simulink model "sampleModel280"  (R2021b)
settings: Solver=VariableStepAuto  StartTime=0.0  StopTime=10.0  RelTol=1e-3
undefined symbols (not defined in the file or in its folder): DiscIntNeverNeededParam, Newton, Raphson
libraries: simulink x14, slpidlib x1
settings Model: Creator=user  LastModifiedBy=user

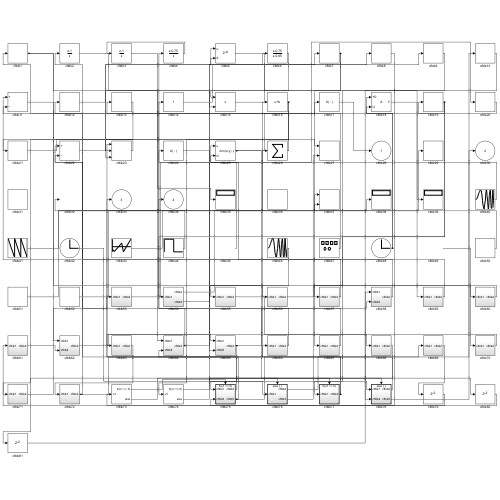
[thumbnail: Simulink's stored preview of the top-level diagram]
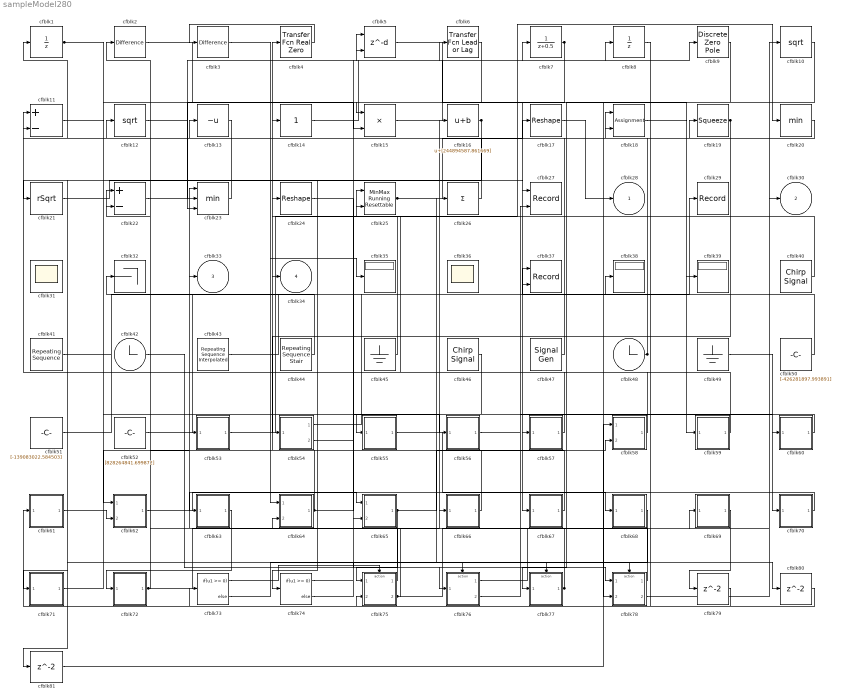
== system sampleModel280 ==
  cfblk1 : UnitDelay  HasFrameUpgradeWarning=on
  cfblk10 : Sqrt  SaturateOnIntegerOverflow=on
  cfblk11 : Sum  Inputs=+-
  cfblk12 : Sqrt  SaturateOnIntegerOverflow=on
  cfblk13 : UnaryMinus
  cfblk14 : simulink/Math Operations/Slider Gain  gain=1  low=0  high=2
  cfblk15 : Product
  cfblk16 : Bias  Bias=[244894587.861669]
  cfblk17 : Reshape
  cfblk18 : Assignment  DiagnosticForDimensions=Warning  IndexOptions=Index vector (dialog)  Indices=1  OutputSizes=1
  cfblk19 : Squeeze
  cfblk2 : simulink/Discrete/Difference  ICPrevInput=0.0  OutMin=[]  OutMax=[]  OutDataTypeStr=Inherit: Inherit via back propagation  OutDataType=fixdt(1, 16)  OutScaling=2^-10  DoSatur=off
  cfblk20 : MinMax
  cfblk21 : Sqrt  Operator=rSqrt  AlgorithmType=Newton-Raphson  SaturateOnIntegerOverflow=on
  cfblk22 : Sum  Inputs=+-
  cfblk23 : MinMax  Inputs=3
  cfblk24 : Reshape
  cfblk25 : simulink/Math Operations/MinMax Running Resettable  Function=min  vinit=0.0
  cfblk26 : Sum  Inputs=+
  cfblk27 : Record  FileSettingsInternal="{\"entries\":[{\"content\":{\"excelSettings\":{\"content\":{},\"type\":\"Streamout.ExcelSettings\"}},\"type\":\"Streamout.FileSettingStorage\",\"uuid\":\"01a86b24-10fd-47b5-8f86-b590ee2283c4\"}],\"packageUris\":[\"http://schema.mathworks.com/mf0/streamout_blocks/R2020a\"],\"version\":\"1.0\"}"  Layout=[1 1]  SignalsInternal="{\"entries\":[{\"content\":{\"signals\":[{\"content\":{\"blockPath\":[\"sampleModel280/cfblk27\"],\"channel\":[],\"dimensions\":[1],\"domain\":\"sampleModel280/cfblk27\",\"lineColor\":\"#a2142f\",\"plots\":[1],\"port\":1,\"sid\":[\"\"],\"signalID\":11869,\"signalName\":\"cfblk21\"},\"type\":\"RecordBlkView.Signal\",\"uuid\":\"a0fc44e3-e2e4-42ff-bb3b-f537f22ba603\"},{\"content\":{\"blockPath\":[\"sampleModel280/cfblk27\"],\"channel\":[],\"dimensions\":[1],\"domain\":\"sampleModel280/cfblk27\",\"lineColor\":\"#139fff\",\"plots\":[1],\"port\":2,\"sid\":[\"\"],\"signalID\":11873,\"signalName\":\"cfblk76:2\"},\"type\":\"RecordBlkView.Signal\",\"uuid\":\"77bcc749-ff83-4f0f-aafb-09d3bf5905dd\"}]},\"type\":\"RecordBlkView.InputSignals\",\"uuid\":\"96dfc8e1-6c66-4ba5-9853-10110527c52c\"}],\"packageUris\":[\"http://schema.mathworks.com/mf0/streamout_blocks/R2020a\"],\"version\":\"1.0\"}"  VisualizationBindings="{\"xyplotplugin\":{\"info\":[{\"series\":[{\"bindingParametersList\":[{\"parameter\":\"X-Axis\",\"signalID\":11869,\"signalName\":\"cfblk21\"},{\"parameter\":\"Y-Axis\",\"signalID\":11873,\"signalName\":\"cfblk76:2\"}],\"seriesID\":38376}],\"subplotID\":1}]}}"  CompatibilityTag=XY
  cfblk29 : Record  FileSettingsInternal="{\"entries\":[{\"content\":{\"excelSettings\":{\"content\":{},\"type\":\"Streamout.ExcelSettings\"}},\"type\":\"Streamout.FileSettingStorage\",\"uuid\":\"e8b19c5e-8c0f-47fc-b4c9-298200dd95d7\"}],\"packageUris\":[\"http://schema.mathworks.com/mf0/streamout_blocks/R2020a\"],\"version\":\"1.0\"}"  SignalsInternal="{\"entries\":[{\"content\":{\"signals\":[{\"content\":{\"blockPath\":[\"sampleModel280/cfblk29\"],\"channel\":[],\"dimensions\":[1],\"domain\":\"sampleModel280/cfblk29\",\"lineColor\":\"#edb120\",\"plots\":[1],\"port\":1,\"sid\":[\"\"],\"signalID\":11881,\"signalName\":\"cfblk51\"},\"type\":\"RecordBlkView.Signal\",\"uuid\":\"65e0956e-956d-4622-b740-1f07b225f85c\"}]},\"type\":\"RecordBlkView.InputSignals\",\"uuid\":\"866c25ee-dbf6-4b5f-85e6-0975c442b7af\"}],\"packageUris\":[\"http://schema.mathworks.com/mf0/streamout_blocks/R2020a\"],\"version\":\"1.0\"}"  VisualizationBindings="{\"sparklinesplugin\":{\"info\":[{\"bindingParametersList\":[],\"subplotID\":1}]}}"
  cfblk3 : simulink/Discrete/Difference  ICPrevInput=0.0  OutMin=[]  OutMax=[]  OutDataTypeStr=Inherit: Inherit via back propagation  OutDataType=fixdt(1, 16)  OutScaling=2^-10  DoSatur=off
  cfblk31 : Scope
      settings: Floating=on
  cfblk32 : Terminator
  cfblk35 : Display
  cfblk36 : Scope
      settings: Floating=on
  cfblk37 : Record  FileSettingsInternal="{\"entries\":[{\"content\":{\"excelSettings\":{\"content\":{},\"type\":\"Streamout.ExcelSettings\"}},\"type\":\"Streamout.FileSettingStorage\",\"uuid\":\"e62b4aea-36b7-4c87-85d7-a4ab9cb59138\"}],\"packageUris\":[\"http://schema.mathworks.com/mf0/streamout_blocks/R2020a\"],\"version\":\"1.0\"}"  Layout=[1 1]  SignalsInternal="{\"entries\":[{\"content\":{\"signals\":[{\"content\":{\"blockPath\":[\"sampleModel280/cfblk37\"],\"channel\":[],\"dimensions\":[1],\"domain\":\"sampleModel280/cfblk37\",\"lineColor\":\"#a2142f\",\"plots\":[1],\"port\":1,\"sid\":[\"\"],\"signalID\":11885,\"signalName\":\"cfblk43\"},\"type\":\"RecordBlkView.Signal\",\"uuid\":\"4226a702-03e0-4b16-abca-3234c63018e1\"},{\"content\":{\"blockPath\":[\"sampleModel280/cfblk37\"],\"channel\":[],\"dimensions\":[1],\"domain\":\"sampleModel280/cfblk37\",\"lineColor\":\"#139fff\",\"plots\":[1],\"port\":2,\"sid\":[\"\"],\"signalID\":11889,\"signalName\":\"cfblk50\"},\"type\":\"RecordBlkView.Signal\",\"uuid\":\"55b215cc-d555-4d8f-b13f-ef35d573dbbd\"}]},\"type\":\"RecordBlkView.InputSignals\",\"uuid\":\"d3c2a2c5-2de7-407e-9157-1018b6e42a97\"}],\"packageUris\":[\"http://schema.mathworks.com/mf0/streamout_blocks/R2020a\"],\"version\":\"1.0\"}"  VisualizationBindings="{\"xyplotplugin\":{\"info\":[{\"series\":[{\"bindingParametersList\":[{\"parameter\":\"X-Axis\",\"signalID\":11885,\"signalName\":\"cfblk43\"},{\"parameter\":\"Y-Axis\",\"signalID\":11889,\"signalName\":\"cfblk50\"}],\"seriesID\":28925}],\"subplotID\":1}]}}"  CompatibilityTag=XY
  cfblk38 : Display
  cfblk39 : Display
  cfblk4 : simulink/Discrete/Transfer Fcn Real Zero  ZeroZ=0.75  ICPrevInput=0.0  DoSatur=off
      settings: SourceProductBaseCode=SL
  cfblk40 : simulink/Sources/Chirp Signal  f1=[477583071.067130]  T=[170289565.158624]  f2=[-132189540.561952]
  cfblk41 : simulink/Sources/Repeating Sequence  rep_seq_t=[0 2]  rep_seq_y=[470306380.096808, -725988435.533882]
  cfblk42 : Clock
  cfblk43 : simulink/Sources/Repeating Sequence Interpolated  OutValues=[-280109527.984477, -640686721.339378, 480149620.737201, -658559004.004570, 983301595.274376]  TimeValues=[0 0.1 0.5 0.6 1].'  LookUpMeth=Interpolation-Use End Values  tsamp=0.01  OutMin=[]  OutMax=[]  OutDataTypeStr=double  OutputDataTypeScalingMode=double  OutDataType=fixdt(0,8)  OutScaling=2^-10
  cfblk44 : simulink/Sources/Repeating Sequence Stair  OutValues=[152099642.248450, 137848680.236196]  tsamp=-1  OutMin=[]  OutMax=[]  OutDataTypeStr=double  OutputDataTypeScalingMode=double  OutDataType=fixdt(0,8)  ConRadixGroup=Best Precision: Vector-wise  OutScaling=2^-12
  cfblk45 : Ground
  cfblk46 : simulink/Sources/Chirp Signal  f1=[-254697657.951645]  T=[-710962001.298007]  f2=[-290174974.004187]
  cfblk47 : SignalGenerator  WaveForm=square  Amplitude=[315229153.492773]  Units=rad/sec
  cfblk48 : Clock
  cfblk49 : Ground
  cfblk5 : Delay  DelayLengthSource=Input port  SampleTime=1
      settings: InputPortMap=u0,p1
  cfblk50 : Constant  Value=[-426281897.993891]  SampleTime=1
  cfblk51 : Constant  Value=[-139083022.584503]  SampleTime=1
  cfblk52 : Constant  Value=[828264841.699872]  SampleTime=1
  cfblk53 : Subsystem
  cfblk54 : Subsystem
  cfblk55 : Subsystem
  cfblk56 : Subsystem
  cfblk57 : Subsystem
  cfblk58 : Subsystem
  cfblk59 : Subsystem
  cfblk6 : simulink/Discrete/Transfer Fcn Lead or Lag  PoleZ=0.95  ZeroZ=0.75  ICPrevOutput=0.0  ICPrevInput=0.0  DoSatur=off
      settings: SourceProductBaseCode=SL
  cfblk60 : Subsystem
  cfblk61 : Subsystem
  cfblk62 : Subsystem
  cfblk63 : Subsystem
  cfblk64 : Subsystem
  cfblk65 : Subsystem
  cfblk66 : Subsystem
  cfblk67 : Subsystem
  cfblk68 : Subsystem
  cfblk69 : Subsystem
  cfblk7 : DiscreteTransferFcn  SampleTime=1
  cfblk70 : Subsystem
  cfblk71 : Subsystem
  cfblk72 : Subsystem
  cfblk73 : If  IfExpression=u1 >= 0  SampleTime=1
  cfblk74 : If  IfExpression=u1 >= 0  SampleTime=1
  cfblk75 : Subsystem  TreatAsAtomicUnit=on
  cfblk76 : Subsystem  TreatAsAtomicUnit=on
  cfblk77 : Subsystem  TreatAsAtomicUnit=on
  cfblk78 : Subsystem  TreatAsAtomicUnit=on
  cfblk79 : Delay  SampleTime=1
  cfblk8 : UnitDelay  HasFrameUpgradeWarning=on
  cfblk80 : Delay  SampleTime=1
  cfblk81 : Delay  SampleTime=1
  cfblk9 : DiscreteZeroPole  Poles=[0 0.5]  Gain=1
  cfblk28 : Outport
  cfblk30 : Outport  Port=2
  cfblk33 : Outport  Port=3
  cfblk34 : Outport  Port=4
  wires:
  cfblk26/1 -> cfblk13/1
  cfblk78/1(cfblk2) -> cfblk23/1
  cfblk17/1 -> cfblk28/1
  cfblk7/1 -> cfblk67/1(cfblk1), cfblk15/1
  cfblk53/1(cfblk2) -> cfblk20/1
  cfblk15/1 -> cfblk8/1
  cfblk64/1(cfblk2) -> cfblk4/1, cfblk9/1
  cfblk42/1 -> cfblk78/1(cfblk1)
  cfblk62/1(cfblk2) -> cfblk65/1(cfblk1)
  cfblk44/1 -> cfblk32/1
  cfblk75/1(cfblk2) -> cfblk33/1
  cfblk20/1 -> cfblk19/1
  cfblk52/1 -> cfblk14/1
  cfblk63/1(cfblk2) -> cfblk72/1(cfblk1)
  cfblk8/1 -> cfblk61/1(cfblk1)
  cfblk54/1(cfblk2) -> cfblk38/1
  cfblk65/1(cfblk2) -> cfblk75/1(cfblk1), cfblk58/2(cfblk5)
  cfblk58/1(cfblk2) -> cfblk12/1
  cfblk13/1 -> cfblk71/1(cfblk1)
  cfblk2/1 -> cfblk64/1(cfblk1)
  cfblk21/1 -> cfblk27/1
  cfblk67/1(cfblk2) -> cfblk34/1
  cfblk3/1 -> cfblk35/1
  cfblk57/1(cfblk2) -> cfblk25/1
  cfblk25/1 -> cfblk17/1, cfblk80/1
  cfblk19/1 -> cfblk54/1(cfblk1), cfblk18/2, cfblk77/1(cfblk1)
  cfblk70/1(cfblk2) -> cfblk63/1(cfblk1)
  cfblk72/1(cfblk2) -> cfblk16/1, cfblk22/2
  cfblk71/1(cfblk2) -> cfblk53/1(cfblk1)
  cfblk4/1 -> cfblk3/1
  cfblk59/1(cfblk2) -> cfblk11/1
  cfblk55/1(cfblk2) -> cfblk68/1(cfblk1)
  cfblk16/1 -> cfblk74/1, cfblk23/3
  cfblk10/1 -> cfblk78/2(cfblk4)
  cfblk40/1 -> cfblk25/2
  cfblk11/1 -> cfblk56/1(cfblk1)
  cfblk49/1 -> cfblk70/1(cfblk1)
  cfblk9/1 -> cfblk57/1(cfblk1)
  cfblk22/1 -> cfblk5/1
  cfblk45/1 -> cfblk24/1
  cfblk66/1(cfblk2) -> cfblk22/1
  cfblk75/2(cfblk5) -> cfblk69/1(cfblk1), cfblk64/2(cfblk4)
  cfblk5/1 -> cfblk59/1(cfblk1)
  cfblk23/1 -> cfblk21/1
  cfblk14/1 -> cfblk7/1
  cfblk51/1 -> cfblk29/1
  cfblk60/1(cfblk2) -> cfblk55/1(cfblk1)
  cfblk47/1 -> cfblk11/2
  cfblk56/1(cfblk2) -> cfblk60/1(cfblk1)
  cfblk24/1 -> cfblk76/1(cfblk1)
  cfblk46/1 -> cfblk65/2(cfblk5)
  cfblk54/2(cfblk5) -> cfblk6/1
  cfblk41/1 -> cfblk26/1
  cfblk43/1 -> cfblk37/1
  cfblk18/1 -> cfblk39/1
  cfblk1/1 -> cfblk62/1(cfblk1), cfblk15/2
  cfblk61/1(cfblk2) -> cfblk62/2(cfblk4)
  cfblk78/2(cfblk5) -> cfblk30/1
  cfblk50/1 -> cfblk37/2
  cfblk48/1 -> cfblk1/1, cfblk18/1
  cfblk6/1 -> cfblk23/2
  cfblk77/1(cfblk2) -> cfblk2/1, cfblk66/1(cfblk1)
  cfblk12/1 -> cfblk5/2
  cfblk76/1(cfblk2) -> cfblk10/1
  cfblk76/2(cfblk3) -> cfblk27/2
  cfblk73/1 -> cfblk75/Action
  cfblk73/2 -> cfblk76/Action
  cfblk74/1 -> cfblk77/Action
  cfblk74/2 -> cfblk78/Action
  cfblk69/1(cfblk2) -> cfblk79/1
  cfblk79/1 -> cfblk75/2(cfblk4)
  cfblk80/1 -> cfblk73/1
  cfblk68/1(cfblk2) -> cfblk81/1
  cfblk81/1 -> cfblk58/1(cfblk1)

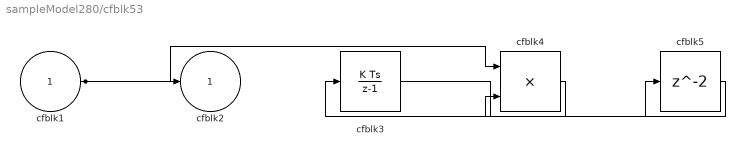
== system sampleModel280/cfblk53 ==
  cfblk1 : Inport
  cfblk3 : DiscreteIntegrator  ICPrevOutput=DiscIntNeverNeededParam  ICPrevScaledInput=DiscIntNeverNeededParam
  cfblk4 : Product  Inputs=**
  cfblk5 : Delay  SampleTime=1
  cfblk2 : Outport
  wires:
  cfblk1/1 -> cfblk4/1, cfblk2/1
  cfblk4/1 -> cfblk3/1
  cfblk3/1 -> cfblk5/1
  cfblk5/1 -> cfblk4/2

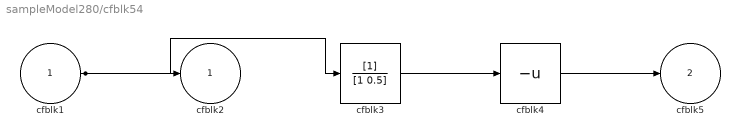
== system sampleModel280/cfblk54 ==
  cfblk1 : Inport
  cfblk3 : DiscreteFilter  SampleTime=1
  cfblk4 : UnaryMinus
  cfblk2 : Outport
  cfblk5 : Outport  Port=2
  wires:
  cfblk1/1 -> cfblk3/1, cfblk2/1
  cfblk3/1 -> cfblk4/1
  cfblk4/1 -> cfblk5/1

== system sampleModel280/cfblk55 ==
  cfblk1 : Inport
  cfblk3 : Assignment  DiagnosticForDimensions=Warning  IndexOptions=Index vector (dialog)  Indices=1  OutputSizes=1
  cfblk2 : Outport
  wires:
  cfblk1/1 -> cfblk3/1, cfblk3/2
  cfblk3/1 -> cfblk2/1

== system sampleModel280/cfblk56 ==
  cfblk1 : Inport
  cfblk3 : slpidlib/PID Controller  Controller=PID  Form=Parallel  TimeDomain=Discrete-time  UseExternalTs=off  SampleTime=1  IntegratorMethod=Forward Euler  FilterMethod=Forward Euler  ControllerParametersSource=internal  P=1  I=1  D=0  UseFilter=on  N=100  TunerSelectOption=Transfer Function Based (PID Tuner App)  InitialConditionSource=internal  InitialConditionForIntegrator=0  InitialConditionForFilter=0  DifferentiatorICPrevScaledInput=0  ExternalReset=none  TrackingMode=off  Kt=1  LimitOutput=off  SatLimitsSource=internal  UpperSaturationLimit=inf  LowerSaturationLimit=-inf  LinearizeAsGain=off  AntiWindupMode=none  Kb=1  POutMin=[]  POutMax=[]  IOutMin=[]  IOutMax=[]  DOutMin=[]  DOutMax=[]  NOutMin=[]  NOutMax=[]  SumOutMin=[]  SumOutMax=[]  SaturationOutMin=[]  SaturationOutMax=[]  PParamMin=[]  PParamMax=[]  IParamMin=[]  IParamMax=[]  DParamMin=[]  DParamMax=[]  NParamMin=[]  NParamMax=[]  KbParamMin=[]  KbParamMax=[]  KtParamMin=[]  KtParamMax=[]  KbOutMin=[]  KbOutMax=[]  KtOutMin=[]  KtOutMax=[]  IntegratorOutMin=[]  IntegratorOutMax=[]  FilterOutMin=[]  FilterOutMax=[]  SumI1OutMin=[]  SumI1OutMax=[]  SumI2OutMin=[]  SumI2OutMax=[]  SumI3OutMin=[]  SumI3OutMax=[]  SumI4OutMin=[]  SumI4OutMax=[]  SumDOutMin=[]  SumDOutMax=[]  DifferentiatorOutMin=[]  DifferentiatorOutMax=[]  FilterDiffOutCoefMin=[]  FilterDiffOutCoefMax=[]  ReciprocalOutMin=[]  ReciprocalOutMax=[]  SumDenOutMin=[]  SumDenOutMax=[]  SumNumOutMin=[]  SumNumOutMax=[]  DivideOutMin=[]  DivideOutMax=[]  UdiffTsProdOutMin=[]  UdiffTsProdOutMax=[]  NTsProdOutMin=[]  NTsProdOutMax=[]  UintegralTsProdOutMin=[]  UintegralTsProdOutMax=[]  UngainTsProdOutMin=[]  UngainTsProdOutMax=[]  IntegratorContinuousStateAttributes=''  IntegratorStateMustResolveToSignalObject=off  IntegratorRTWStateStorageClass=Auto  FilterContinuousStateAttributes=''  FilterStateMustResolveToSignalObject=off  FilterRTWStateStorageClass=Auto  ParallelPVariant=InternalParameters  IdealPVariant=Disabled  IVariant=InternalParameters  DVariant=InternalParameters  IntegratorVariant=Discrete  SatVariant=Disabled  AWVariant=Passthrough  PCopyVariant=Disabled  TRVariant=Disabled  FdbkBlocksVariant=Forward  IdealPFdbkVariant=Disabled  SatFdbkVariant=Disabled  DerivativeFilterVariant=ForwardEulerFilter  NVariant=InternalParameters  NCopyVariant=Disabled  FilterICVariant=InternalICsFilter  IntegratorICVariant=InternalICs  ExternalResetVariant=Disabled  TRSumVariant=Passthrough  SumFdbkVariant=Disabled  SumVariant=Sum_PID  TsampFilterVariant=InternalTs  TsampNgainVariant=Passthrough  TsampIntegralVariant=Passthrough  ExternalSaturationOutDataTypeStr=Inherit: Same as second input
  cfblk4 : Product  Inputs=*
  cfblk2 : Outport
  wires:
  cfblk4/1 -> cfblk2/1
  cfblk3/1 -> cfblk4/1
  cfblk1/1 -> cfblk3/1

== system sampleModel280/cfblk57 ==
  cfblk1 : Inport
  cfblk3 : DotProduct  InputSameDT=on  OutDataTypeStr=Inherit: Inherit via internal rule
  cfblk2 : Outport
  wires:
  cfblk1/1 -> cfblk3/1, cfblk3/2
  cfblk3/1 -> cfblk2/1

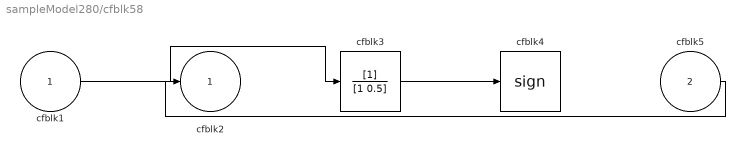
== system sampleModel280/cfblk58 ==
  cfblk1 : Inport
  cfblk5 : Inport  Port=2
  cfblk3 : DiscreteFilter  SampleTime=1
  cfblk4 : Signum
  cfblk2 : Outport
  wires:
  cfblk3/1 -> cfblk4/1
  cfblk1/1 -> cfblk3/1
  cfblk5/1 -> cfblk2/1

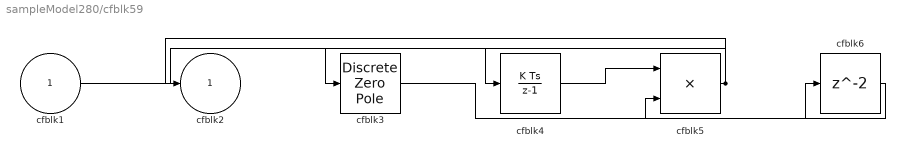
== system sampleModel280/cfblk59 ==
  cfblk1 : Inport
  cfblk3 : DiscreteZeroPole  Poles=[0 0.5]  Gain=1
  cfblk4 : DiscreteIntegrator  ICPrevOutput=DiscIntNeverNeededParam  ICPrevScaledInput=DiscIntNeverNeededParam
  cfblk5 : Product  Inputs=**
  cfblk6 : Delay  SampleTime=1
  cfblk2 : Outport
  wires:
  cfblk1/1 -> cfblk4/1
  cfblk4/1 -> cfblk5/1
  cfblk5/1 -> cfblk2/1, cfblk3/1
  cfblk3/1 -> cfblk6/1
  cfblk6/1 -> cfblk5/2

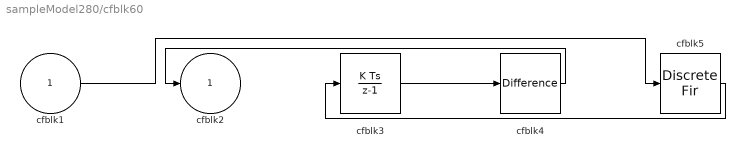
== system sampleModel280/cfblk60 ==
  cfblk1 : Inport
  cfblk3 : DiscreteIntegrator  ICPrevOutput=DiscIntNeverNeededParam  ICPrevScaledInput=DiscIntNeverNeededParam
  cfblk4 : simulink/Discrete/Difference  ICPrevInput=0.0  OutMin=[]  OutMax=[]  OutDataTypeStr=Inherit: Inherit via back propagation  OutDataType=fixdt(1, 16)  OutScaling=2^-10  DoSatur=off
  cfblk5 : DiscreteFir  SampleTime=1
  cfblk2 : Outport
  wires:
  cfblk3/1 -> cfblk4/1
  cfblk4/1 -> cfblk2/1
  cfblk5/1 -> cfblk3/1
  cfblk1/1 -> cfblk5/1

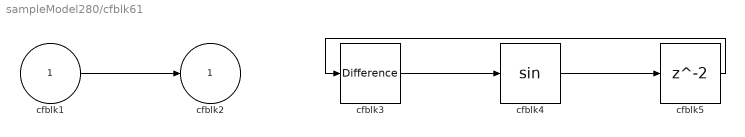
== system sampleModel280/cfblk61 ==
  cfblk1 : Inport
  cfblk3 : simulink/Discrete/Difference  ICPrevInput=0.0  OutMin=[]  OutMax=[]  OutDataTypeStr=Inherit: Inherit via back propagation  OutDataType=fixdt(1, 16)  OutScaling=2^-10  DoSatur=off
  cfblk4 : Trigonometry
  cfblk5 : Delay  SampleTime=1
  cfblk2 : Outport
  wires:
  cfblk3/1 -> cfblk4/1
  cfblk1/1 -> cfblk2/1
  cfblk4/1 -> cfblk5/1
  cfblk5/1 -> cfblk3/1

== system sampleModel280/cfblk62 ==
  cfblk1 : Inport
  cfblk4 : Inport  Port=2
  cfblk3 : Constant  Value=[452989492.075059]  SampleTime=1
  cfblk2 : Outport
  wires:
  cfblk4/1 -> cfblk2/1

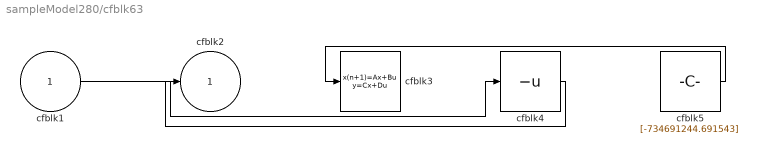
== system sampleModel280/cfblk63 ==
  cfblk1 : Inport
  cfblk3 : DiscreteStateSpace
  cfblk4 : UnaryMinus
  cfblk5 : Constant  Value=[-734691244.691543]  SampleTime=1
  cfblk2 : Outport
  wires:
  cfblk5/1 -> cfblk3/1
  cfblk1/1 -> cfblk4/1
  cfblk4/1 -> cfblk2/1

== system sampleModel280/cfblk64 ==
  cfblk1 : Inport
  cfblk4 : Inport  Port=2
  cfblk3 : DiscreteIntegrator  ICPrevOutput=DiscIntNeverNeededParam  ICPrevScaledInput=DiscIntNeverNeededParam
  cfblk2 : Outport
  wires:
  cfblk4/1 -> cfblk3/1
  cfblk1/1 -> cfblk2/1

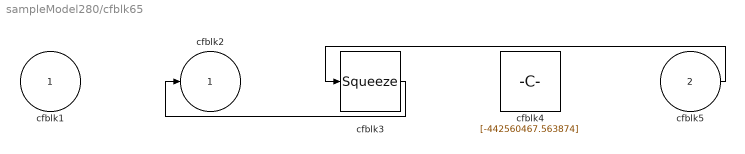
== system sampleModel280/cfblk65 ==
  cfblk1 : Inport
  cfblk5 : Inport  Port=2
  cfblk3 : Squeeze
  cfblk4 : Constant  Value=[-442560467.563874]  SampleTime=1
  cfblk2 : Outport
  wires:
  cfblk5/1 -> cfblk3/1
  cfblk3/1 -> cfblk2/1

== system sampleModel280/cfblk66 ==
  cfblk1 : Inport
  cfblk3 : Sin  TimeSource=Use external signal  SampleTime=0
  cfblk2 : Outport
  wires:
  cfblk3/1 -> cfblk2/1
  cfblk1/1 -> cfblk3/1

== system sampleModel280/cfblk67 ==
  cfblk1 : Inport
  cfblk3 : Delay  DelayLengthSource=Input port  SampleTime=1
      settings: InputPortMap=u0,p1
  cfblk4 : Constant  Value=[745806801.382986]  SampleTime=1
  cfblk2 : Outport
  wires:
  cfblk1/1 -> cfblk2/1
  cfblk4/1 -> cfblk3/1, cfblk3/2

== system sampleModel280/cfblk68 ==
  cfblk1 : Inport
  cfblk3 : Constant  Value=[412080624.706913]  SampleTime=1
  cfblk2 : Outport
  wires:
  cfblk1/1 -> cfblk2/1

== system sampleModel280/cfblk69 ==
  cfblk1 : Inport
  cfblk3 : simulink/Math Operations/Slider Gain  gain=1  low=0  high=2
  cfblk2 : Outport
  wires:
  cfblk1/1 -> cfblk3/1
  cfblk3/1 -> cfblk2/1

== system sampleModel280/cfblk70 ==
  cfblk1 : Inport
  cfblk3 : Trigonometry
  cfblk4 : ComplexToMagnitudeAngle
  cfblk5 : Constant  Value=[372575588.669892]  SampleTime=1
  cfblk2 : Outport
  wires:
  cfblk1/1 -> cfblk4/1
  cfblk5/1 -> cfblk3/1
  cfblk4/1 -> cfblk2/1

== system sampleModel280/cfblk71 ==
  cfblk1 : Inport
  cfblk3 : DiscreteIntegrator  ICPrevOutput=DiscIntNeverNeededParam  ICPrevScaledInput=DiscIntNeverNeededParam
  cfblk4 : Sum
  cfblk5 : Delay  SampleTime=1
  cfblk2 : Outport
  wires:
  cfblk3/1 -> cfblk2/1, cfblk5/1
  cfblk4/1 -> cfblk3/1
  cfblk1/1 -> cfblk4/1
  cfblk5/1 -> cfblk4/2

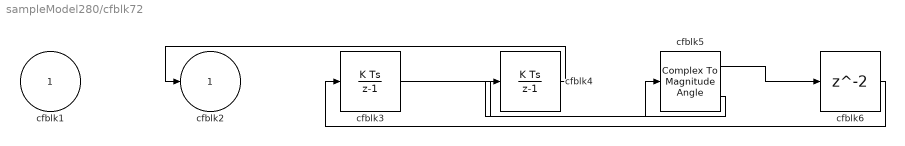
== system sampleModel280/cfblk72 ==
  cfblk1 : Inport
  cfblk3 : DiscreteIntegrator  ICPrevOutput=DiscIntNeverNeededParam  ICPrevScaledInput=DiscIntNeverNeededParam
  cfblk4 : DiscreteIntegrator  ICPrevOutput=DiscIntNeverNeededParam  ICPrevScaledInput=DiscIntNeverNeededParam
  cfblk5 : ComplexToMagnitudeAngle
  cfblk6 : Delay  SampleTime=1
  cfblk2 : Outport
  wires:
  cfblk4/1 -> cfblk2/1
  cfblk3/1 -> cfblk5/1
  cfblk5/2 -> cfblk4/1
  cfblk5/1 -> cfblk6/1
  cfblk6/1 -> cfblk3/1

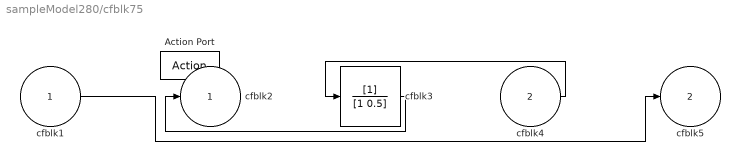
== system sampleModel280/cfblk75 ==
  cfblk1 : Inport
  cfblk4 : Inport  Port=2
  Action Port : ActionPort  ActionPortLabel=if(u1 >= 0)
  cfblk3 : DiscreteFilter
  cfblk2 : Outport
  cfblk5 : Outport  Port=2
  wires:
  cfblk4/1 -> cfblk3/1
  cfblk3/1 -> cfblk2/1
  cfblk1/1 -> cfblk5/1

== system sampleModel280/cfblk76 ==
  cfblk1 : Inport
  Action Port : ActionPort  ActionPortLabel=else
  cfblk2 : Outport
  cfblk3 : Outport  Port=2
  wires:
  cfblk1/1 -> cfblk3/1, cfblk2/1

== system sampleModel280/cfblk77 ==
  cfblk1 : Inport
  Action Port : ActionPort  ActionPortLabel=if(u1 >= 0)
  cfblk3 : DiscreteStateSpace  SampleTime=-1
  cfblk2 : Outport
  wires:
  cfblk1/1 -> cfblk2/1, cfblk3/1

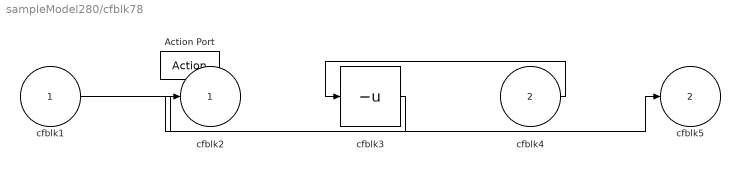
== system sampleModel280/cfblk78 ==
  cfblk1 : Inport
  cfblk4 : Inport  Port=2
  Action Port : ActionPort  ActionPortLabel=else
  cfblk3 : UnaryMinus
  cfblk2 : Outport
  cfblk5 : Outport  Port=2
  wires:
  cfblk1/1 -> cfblk5/1
  cfblk4/1 -> cfblk3/1
  cfblk3/1 -> cfblk2/1
